simulink model "Example_8_4a"  (R2014a)
settings: Solver=FixedStepDiscrete  SolverMode=SingleTasking  StartTime=0.0  StopTime=10  FixedStep=1  RelTol=1e-3
settings Model: Creator=Lee Edwards  LastModifiedBy=Lee
settings DataIOCC: SignalLoggingSaveFormat=ModelDataLogs  SaveOutput=off  SignalLogging=off  SaveTime=off
settings OptimizationCC: ExpressionDepthLimit=2147483647
settings DebuggingCC: AlgebraicLoopMsg=error  UnderspecifiedInitializationDetection=Classic  SingleTaskRateTransMsg=error  FcnCallInpInsideContextMsg=UseLocalSettings  StateNameClashWarn=warning
settings GRTTargetCC: CombineOutputUpdateFcns=off  GRTInterface=on

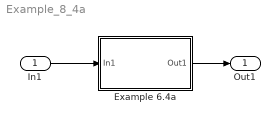
== system Example_8_4a ==
  In1 : Inport
  Example 6.4a : Subsystem
  Out1 : Outport
  wires:
  Example 6.4a/1(Out1) -> Out1/1
  In1/1 -> Example 6.4a/1(In1)

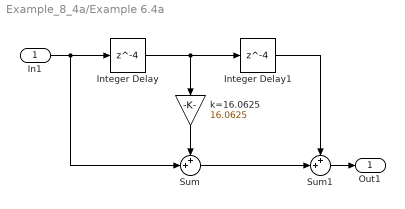
== system Example_8_4a/Example 6.4a ==
  In1 : Inport
  Integer Delay : Delay  DelayLength=4  InputProcessing=Inherited
  Integer Delay1 : Delay  DelayLength=4  InputProcessing=Inherited
  Sum : Sum  Inputs=++|
  Sum1 : Sum  Inputs=++|
  k=16.0625 : Gain  Gain=16.0625
  Out1 : Outport
  wires:
  Integer Delay/1 -> k=16.0625/1, Integer Delay1/1
  In1/1 -> Integer Delay/1, Sum/2
  Integer Delay1/1 -> Sum1/1
  k=16.0625/1 -> Sum/1
  Sum/1 -> Sum1/2
  Sum1/1 -> Out1/1
